simulink model "Lab5_1"  (R2016a)
settings: Solver=FixedStepDiscrete  StartTime=0.0  StopTime=10.0  RelTol=1e-3
undefined symbols (not defined in the file or in its folder): Enum_dataType
libraries: simulink x2
settings Model: Creator=NoteBook  LastModifiedBy=NoteBook
settings OptimizationCC: DefaultParameterBehavior=Inlined  EnableMemcpy=off  OptimizeModelRefInitCode=on  LifeSpan=1
settings DebuggingCC: UnderspecifiedInitializationDetection=Classic  MergeDetectMultiDrivingBlocksExec=none
settings ModelReferenceCC: PropagateSignalLabelsOutOfModel=off
settings RTWCC: SystemTargetFile=ert.tlc  GenCodeOnly=on  TemplateMakefile=ert_default_tmf  GenerateReport=on  IncludeHyperlinkInReport=on  LaunchReport=on  GenerateTraceInfo=on  GenerateTraceReport=on  GenerateTraceReportSl=on  GenerateTraceReportSf=on  GenerateTraceReportEml=on
settings CodeAppCC: ForceParamTrailComments=on  IgnoreCustomStorageClasses=off  OperatorAnnotations=on  SimulinkDataObjDesc=on  SFDataObjDesc=on  MATLABFcnDesc=on  InsertBlockDesc=on  MATLABSourceComments=on
settings ERTTargetCC: GenerateSampleERTMain=on  InlinedParameterPlacement=NonHierarchical  ERTCustomFileTemplate=example_file_process.tlc

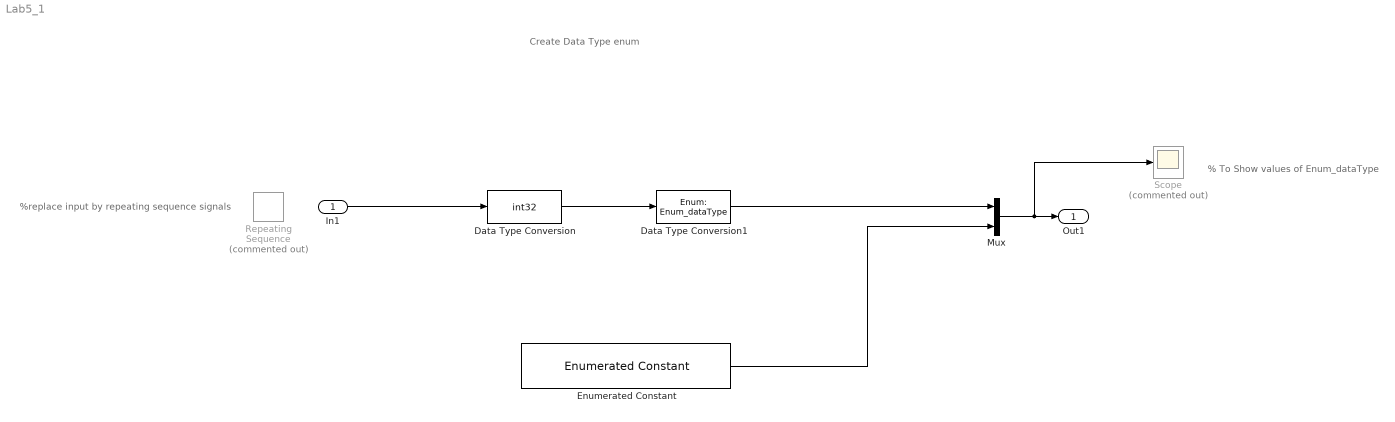
== system Lab5_1 ==
  note: %replace input by repeating sequence signals
  note: Create Data Type enum
  note: % To Show values of Enum_dataType
  In1 : Inport
  Data Type Conversion : DataTypeConversion  OutDataTypeStr=int32
  Data Type Conversion1 : DataTypeConversion  OutDataTypeStr=Enum: Enum_dataType
  Enumerated Constant : simulink/Sources/Enumerated Constant  OutDataTypeStr=Enum: Enum_dataType  Value=Enum_dataType.RCC_enuOK  SampleTime=inf
  Mux : Mux  Inputs=2
  Repeating Sequence : simulink/Sources/Repeating Sequence  Commented=on  rep_seq_t=[0 1 2 3]  rep_seq_y=[0 1 2 3]
  Scope : Scope  Commented=on
  Out1 : Outport
  wires:
  Data Type Conversion/1 -> Data Type Conversion1/1
  Data Type Conversion1/1 -> Mux/1
  Enumerated Constant/1 -> Mux/2
  Mux/1 -> Scope/1, Out1/1
  In1/1 -> Data Type Conversion/1
